simulink model "MGsystem"  (R2024a)
settings: Solver=VariableStepAuto  StartTime=0.0  StopTime=8  RelTol=1e-3
InitFcn:
  | Ts_Control=1e-4;
  | Ts_Power=1e-5;
libraries: spsCurrentMeasurementLib x2, spsThreePhaseSourceLib x1, spsSeriesRLCBranchLib x1, spsGroundLib x1, spsMultimeterLib x1, spsPowerPositiveSequenceLib x1, spsStairGeneratorLib x1, spspowerguiLib x1
settings Model: SimulationMode=accelerator  Creator=nakamura  LastModifiedBy=nakamura

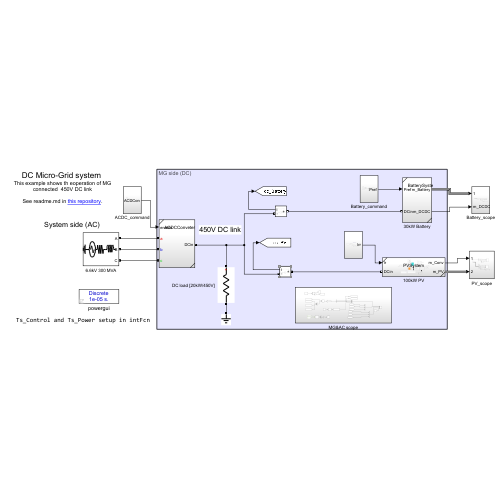
[thumbnail: Simulink's stored preview of the top-level diagram]
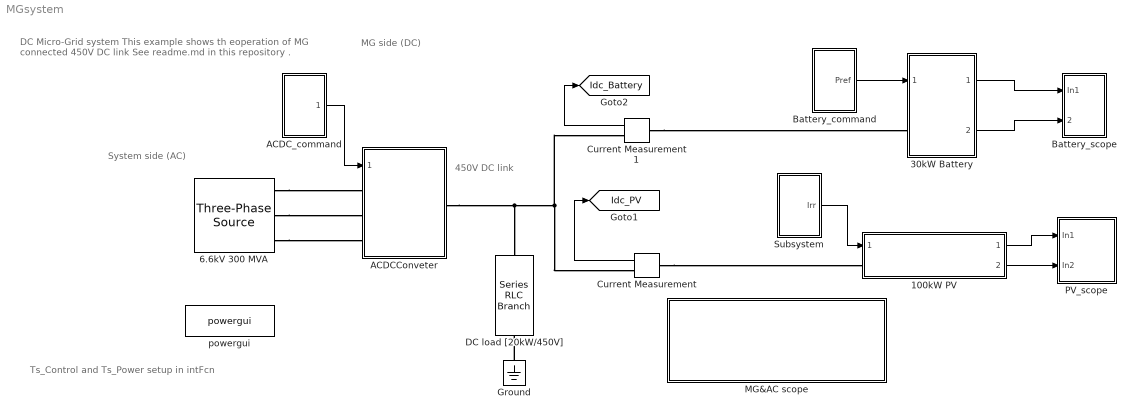
== system MGsystem ==
  note: Ts_Control and Ts_Power setup in intFcn
  note: MG side (DC)
  note: 450V DC link
  note: System side (AC)
  note: DC Micro-Grid system
      | This example shows th eoperation of MG connected 450V DC link
      |
      | See readme.md in this repository .
  100kW PV : Subsystem  ReferencedSubsystem=PVSystem
  30kW Battery : Subsystem  ReferencedSubsystem=BatterySystem
  6.6kV 300 MVA : spsThreePhaseSourceLib/Three-Phase Source  InternalConnection=Yg  VoltagePhases=off  Voltage=6.6e3  PhaseAngle=0  Voltage_phases=[25e3 25e3 25e3]/sqrt(3)  PhaseAngles_phases=[0 -120 +120]  Frequency=60  NonIdealSource=on  SpecifyImpedance=on  Resistance=0.724  Inductance=19.2e-3  ShortCircuitLevel=300e6  BaseVoltage=6.6e3  XRratio=10  BusType=swing  Pref=0  Qref=0  Prefabc=[10e3, 10e3, 10e3]  Qrefabc=[0, 0, 0]  Qmin=-inf  Qmax=inf
  ACDCConveter : Subsystem  ReferencedSubsystem=ACDCConveter
  ACDC_command : Subsystem
  Battery_command : Subsystem
  Battery_scope : Subsystem
  Current Measurement : spsCurrentMeasurementLib/Current Measurement  PhasorSimulation=off  OutputType=Complex  PSBequivalent=0
  Current Measurement1 : spsCurrentMeasurementLib/Current Measurement  PhasorSimulation=off  OutputType=Complex  PSBequivalent=0
  DC load [20kW/450V] : spsSeriesRLCBranchLib/Series RLC Branch  LConnTagsString=__new0  RConnTagsString=__new0  BranchType=R  Resistance=(450^2)/20e3  Inductance=1e-3  SetiL0=off  InitialCurrent=0  Capacitance=1e-6  Setx0=off  InitialVoltage=0  Measurements=Branch voltage and current
  Ground : spsGroundLib/Ground  LConnTagsString=a
  MG&AC scope : Subsystem
  PV_scope : Subsystem
  Subsystem : Subsystem
  powergui : spspowerguiLib/powergui  Priority=2  SimulationMode=Discrete  SampleTime=Ts_Power  frequency=60  Iterations=50  frequencyindice=0  Pbase=100e6  ErrMax=1e-4  UnitsV=kV  UnitsW=MW  buscounter=0  FunctionMessages=off  echomessages=off  EnableUseOfTLC=off  CurrentSourceSwitches=off  DisableSnubberDevices=off  DisableRonSwitches=off  DisableVfSwitches=off  DisplayEquations=off  AutomaticDiscreteSolvers=off  SolverType=Tustin/Backward Euler (TBE)  Interpol=off  ExternalGateDelay=off  methode=off  Ts=100  x0status=blocks  SPID=off  SwTol=0  HookPort=off  NonlinearTolerance=1e-4  nMaxIteration=100  ContinueOnMaxIteration=off  RestoreLinks=warning  ResistiveCurrentMeasurement=off  Frange=logspace(0,3,50)  Ylog=off  Xlog=off  ShowGrid=off  save=off  variable=ZData  structure=VaIa  ZoomFFT=on  StartTime=0.2  cycles=2  DisplayStyle=1  fundamental=60  FreqAxis=off  MaxFrequency=1000  frequencyindicesteady=1  RmsSteady=2  display=off
  tag scope: Idc_Battery=global, Idc_PV=global
  wires:
  100kW PV/1 -> PV_scope/1(In1)
  100kW PV/2 -> PV_scope/2(In2)
  30kW Battery/1 -> Battery_scope/1(In1)
  Current Measurement/1 -> [Idc_PV]
  Current Measurement1/1 -> [Idc_Battery]
  ACDC_command/1(ACDCon) -> ACDCConveter/1
  Battery_command/1(Pref) -> 30kW Battery/1
  Subsystem/1(Irr) -> 100kW PV/1
  30kW Battery/2 -> Battery_scope/2(m_DCDC)
  connections:
  6.6kV 300 MVA/RConn1 -- ACDCConveter/LConn1
  6.6kV 300 MVA/RConn2 -- ACDCConveter/LConn2
  6.6kV 300 MVA/RConn3 -- ACDCConveter/LConn3
  Ground/LConn1 -- DC load [20kW/450V]/RConn1
  ACDCConveter/RConn1 -- Current Measurement1/RConn1 -- Current Measurement/RConn1 -- DC load [20kW/450V]/LConn1
  Current Measurement/LConn1 -- 100kW PV/LConn1
  Current Measurement1/LConn1 -- 30kW Battery/LConn1

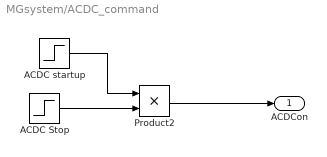
== system MGsystem/ACDC_command ==
  ACDC Stop : Step  Time=4  Before=1  After=0  SampleTime=0
  ACDC startup : Step  Time=0.2  SampleTime=0
  Product2 : Product
  ACDCon : Outport
  wires:
  Product2/1 -> ACDCon/1
  ACDC Stop/1 -> Product2/2
  ACDC startup/1 -> Product2/1

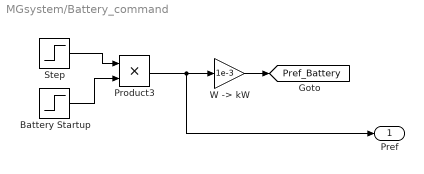
== system MGsystem/Battery_command ==
  Battery Startup : Step  SampleTime=0
  Product3 : Product
  Step : Step  Time=3  Before=-30e3  After=10e3  SampleTime=0
  "W -> kW" : Gain  Gain=1e-3
  Pref : Outport
  tag scope: Pref_Battery=global
  wires:
  Product3/1 -> Pref/1, "W -> kW"/1
  Battery Startup/1 -> Product3/2
  Step/1 -> Product3/1
  "W -> kW"/1 -> [Pref_Battery]

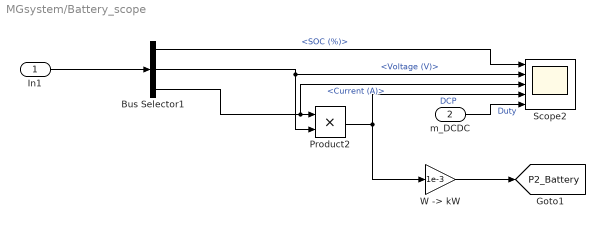
== system MGsystem/Battery_scope ==
  In1 : Inport
  m_DCDC : Inport  Port=2
  Bus Selector1 : BusSelector  OutputSignals=SOC (%),Voltage (V),Current (A)
  Product2 : Product
  Scope2 : Scope  NumInputPorts=5
  "W -> kW" : Gain  Gain=1e-3
  tag scope: P2_Battery=global
  wires:
  In1/1 -> Bus Selector1/1
  Product2/1 -> Scope2/4, "W -> kW"/1  "DCP"
  Bus Selector1/2 -> Product2/2, Scope2/2  "<Voltage (V)>"
  Bus Selector1/3 -> Scope2/3, Product2/1  "<Current (A)>"
  "W -> kW"/1 -> [P2_Battery]
  Bus Selector1/1 -> Scope2/1  "<SOC (%)>"
  m_DCDC/1 -> Scope2/5  "Duty"

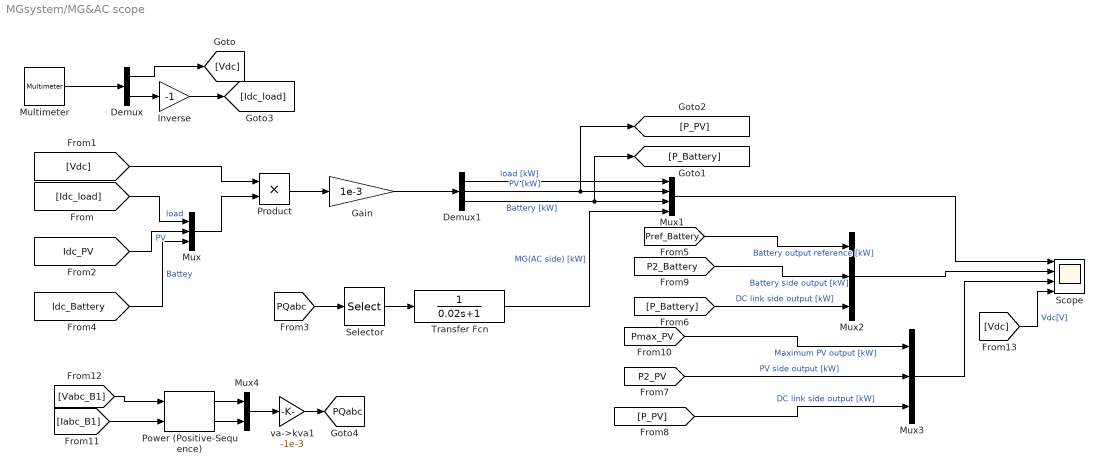
== system MGsystem/MG&AC scope ==
  Demux : Demux  Outputs=2
  Demux1 : Demux  Outputs=3
  Gain : Gain  Gain=1e-3
  Inverse : Gain  Gain=-1
  Multimeter : spsMultimeterLib/Multimeter  L=3  sel=[2 3]  yselected={}  Gain=[1 1]  OutputType=Complex  PlotAtSimulationStop=off  PhasorSimulation=off
  Mux : Mux  Inputs=3
  Mux1 : Mux
  Mux2 : Mux  Inputs=3
  Mux3 : Mux  Inputs=3
  Mux4 : Mux  Inputs=2
  Power (Positive-Sequence) : spsPowerPositiveSequenceLib/Power (Positive-Sequence)  Freq=60  Vinit=[0 0]  Iinit=[0 0]  Ts=Ts_Power
  Product : Product
  Scope : Scope  NumInputPorts=4
  Selector : Selector  InputPortWidth=2  IndexOptions=Index vector (dialog)  Indices=[1]  OutputSizes=1
  Transfer Fcn : TransferFcn  Denominator=[0.02 1]
  va->kva1 : Gain  Gain=-1e-3  SaturateOnIntegerOverflow=on  OutDataTypeStr=Inherit: Same as input  ParamDataTypeStr=Inherit: Same as input
  tag scope: PQabc=global
  wires:
  Demux/2 -> Inverse/1
  Multimeter/1 -> Demux/1
  Demux/1 -> [Vdc]
  [Idc_load] -> Mux/1  "load"
  [Vdc] -> Product/1
  [Idc_PV] -> Mux/2  "PV"
  [Idc_Battery] -> Mux/3  "Battey"
  Mux/1 -> Product/2
  Product/1 -> Gain/1
  Demux1/1 -> Mux1/1  "load [kW]"
  Demux1/2 -> Mux1/2, [P_PV]  "PV [kW]"
  Demux1/3 -> Mux1/3, [P_Battery]  "Battery [kW]"
  [PQabc] -> Selector/1
  Selector/1 -> Transfer Fcn/1
  Gain/1 -> Demux1/1
  Inverse/1 -> [Idc_load]
  Mux1/1 -> Scope/1
  [Pref_Battery] -> Mux2/1  "Battery output reference [kW]"
  [P_Battery] -> Mux2/3  "DC link side output [kW]"
  [P2_PV] -> Mux3/2  "PV side output [kW]"
  [P_PV] -> Mux3/3  "DC link side output [kW]"
  Mux2/1 -> Scope/2
  Mux3/1 -> Scope/3
  [P2_Battery] -> Mux2/2  "Battery side output [kW]"
  [Pmax_PV] -> Mux3/1  "Maximum PV output [kW]"
  [Vabc_B1] -> Power (Positive-Sequence)/1
  Power (Positive-Sequence)/2 -> Mux4/2
  Power (Positive-Sequence)/1 -> Mux4/1
  [Iabc_B1] -> Power (Positive-Sequence)/2
  Mux4/1 -> va->kva1/1
  va->kva1/1 -> [PQabc]
  Transfer Fcn/1 -> Mux1/4  "MG(AC side) [kW]"
  [Vdc] -> Scope/4  "Vdc[V]"

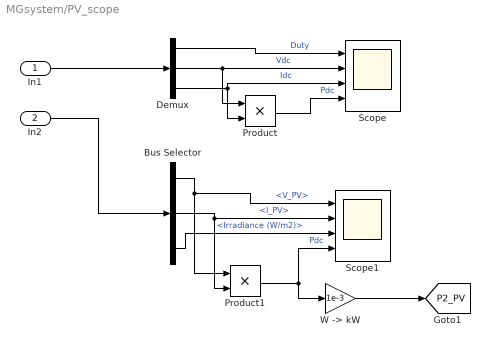
== system MGsystem/PV_scope ==
  In1 : Inport
  In2 : Inport  Port=2
  Bus Selector : BusSelector  OutputSignals=V_PV,I_PV,Irradiance (W/m2)
  Demux : Demux  Outputs=3
  Product : Product
  Product1 : Product
  Scope : Scope  NumInputPorts=4
  Scope1 : Scope  NumInputPorts=4
  "W -> kW" : Gain  Gain=1e-3
  tag scope: P2_PV=global
  wires:
  Demux/1 -> Scope/1  "Duty"
  Bus Selector/1 -> Product1/1, Scope1/1  "<V_PV>"
  Demux/3 -> Product/2, Scope/3  "Idc"
  Bus Selector/2 -> Product1/2, Scope1/2  "<I_PV>"
  Bus Selector/3 -> Scope1/3  "<Irradiance (W/m2)>"
  Product1/1 -> Scope1/4, "W -> kW"/1  "Pdc"
  In1/1 -> Demux/1
  Product/1 -> Scope/4  "Pdc"
  Demux/2 -> Product/1, Scope/2  "Vdc"
  In2/1 -> Bus Selector/1
  "W -> kW"/1 -> [P2_PV]

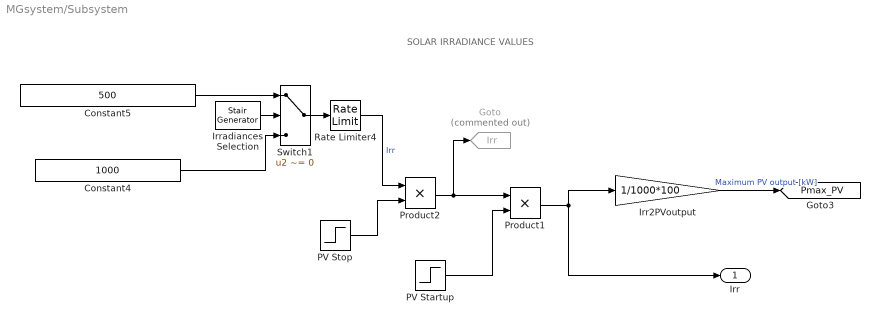
== system MGsystem/Subsystem ==
  note: SOLAR IRRADIANCE VALUES
  Constant4 : Constant  Value=1000
  Constant5 : Constant  Value=500  VectorParams1D=off
  Goto : Goto  Commented=on  GotoTag=Irr  TagVisibility=global
  Irr2PVoutput : Gain  Gain=1/1000*100
  Irradiances Selection : spsStairGeneratorLib/Stair Generator  t=[0, 2, 2.5]  e=[0, 1, 0]  Ts=Ts_Power
  PV Startup : Step  Time=0.5  SampleTime=0
  PV Stop : Step  Time=6  Before=1  After=0  SampleTime=0
  Product1 : Product
  Product2 : Product
  Rate Limiter4 : RateLimiter  RisingSlewLimit=1000*60  FallingSlewLimit=-1000*60  SampleTimeMode=inherited  InitialCondition=1000
  Switch1 : Switch  Criteria=u2 ~= 0  SaturateOnIntegerOverflow=off  InputSameDT=off
  Irr : Outport
  tag scope: Pmax_PV=global
  wires:
  Product1/1 -> Irr/1, Irr2PVoutput/1
  PV Startup/1 -> Product1/2
  Product2/1 -> Goto/1, Product1/1
  Irr2PVoutput/1 -> [Pmax_PV]  "Maximum PV output [kW]"
  PV Stop/1 -> Product2/2
  Irradiances Selection/1 -> Switch1/2
  Constant4/1 -> Switch1/3
  Switch1/1 -> Rate Limiter4/1
  Rate Limiter4/1 -> Product2/1  "Irr"
  Constant5/1 -> Switch1/1
